simulink model "sgMdl_IO601_CAN_HS_Loopback"  (R2024b)
settings: Solver=FixedStepAuto  StartTime=0.0  StopTime=inf  RelTol=1e-3  EnableMultiTasking=on
undefined symbols (not defined in the file): CAN, MESSAGE
libraries: canmsglib x6, speedgoatlib_IO601 x5, slrealtimeutilitieslib x2, simulink x1
Description:
  | IO601 - CAN HS Loopback
settings Model: sg_rtwmakecfg_data=_sglibc_  ModifiedByFormat=Speedgoat  SimulationMode=external  ExtModeTrigDuration=100000  Creator=Speedgoat  LastModifiedBy=Speedgoat
settings SolverCC: ConcurrentTasks=on  AlgebraicLoopSolver=TrustRegion  PositivePriorityOrder=on  InsertRTBMode=Never (minimum delay)
settings DataIOCC: SaveFormat=StructureWithTime  ReturnWorkspaceOutputs=off
settings OptimizationCC: BlockReduction=off  OptimizeBlockIOStorage=off  BufferReuse=off  ReuseModelBlockBuffer=off  GlobalBufferReuse=off  ExpressionFolding=off  LocalBlockOutputs=off
settings DebuggingCC: TasksWithSamePriorityMsg=none  UnconnectedInputMsg=warning  UnconnectedOutputMsg=warning  UnconnectedLineMsg=warning  SFUnexpectedBacktrackingDiag=warning  SFNoUnconditionalDefaultTransitionDiag=warning  SFExecutionAtInitializationDiag=none  ArithmeticOperatorsInVariantConditions=warning
settings HardwareCC: ProdBitPerLong=64  ProdLongLongMode=on  ProdHWDeviceType=Intel->x86-64 (Linux 64)
settings ModelReferenceCC: EnableRefExpFcnMdlSchedulingChecks=on  PropagateSignalLabelsOutOfModel=off
settings SFSimCC: SimUseLocalCustomCode=off  CustomCodeUndefinedFunction=UseInterfaceOnly
settings RTWCC: Description=Speedgoat Real-Time Target Machine  SystemTargetFile=speedgoat.tlc  TemplateMakefile=slrealtime_default_tmf  RTWUseLocalCustomCode=off  Toolchain=Simulink Real-Time Toolchain  BuildConfiguration=Faster Runs  TargetLang=C++  GPUComputeCapability=3.5  DLArmComputeVersion=19.05
settings CodeAppCC: StateflowObjectComments=on
settings SimulinkRealTimeTargetCC: SubcomponentCodeInterfacePackaging=Reusable function  InstructionSetFMA=off  LogToMDFFile=off  SLRTFileLogMaxRuns=10  UseGCCFastMath=on
settings ConfigComp: CovMetricSettings=dw  CovSaveCumulativeToWorkspaceVar=on  CovSaveSingleToWorkspaceVar=on  CovExternalEMLEnable=off  CovBoundaryAbsTol=1.0e-5

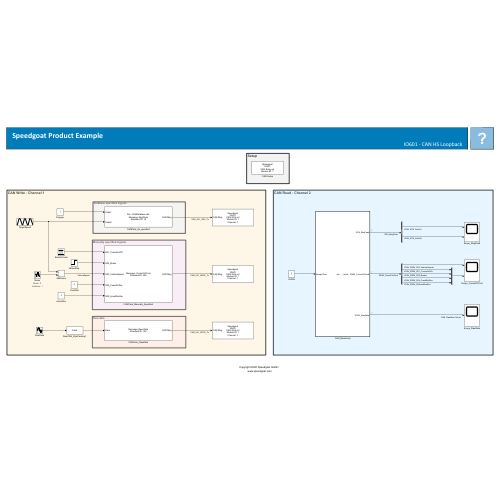
[thumbnail: Simulink's stored preview of the top-level diagram]
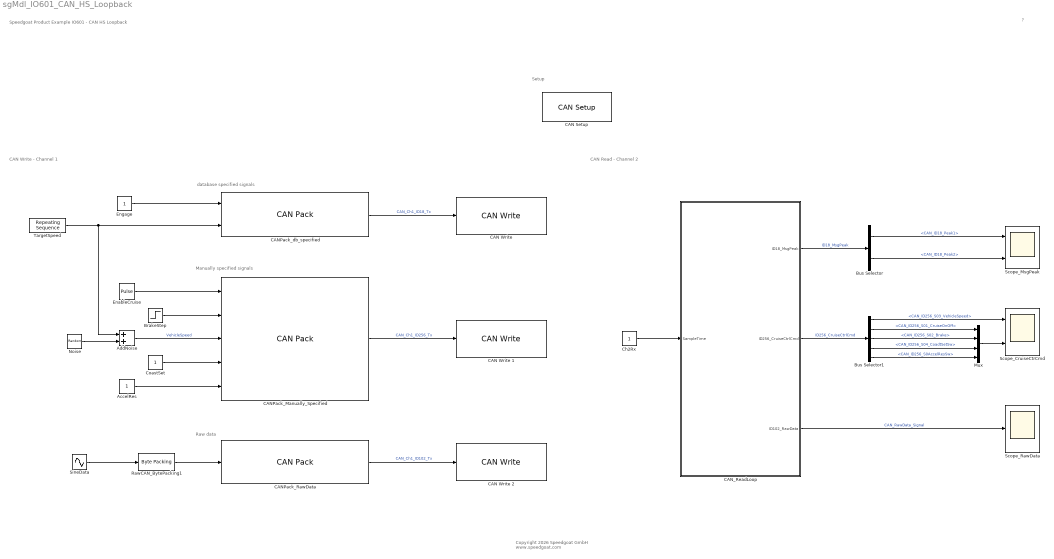
== system sgMdl_IO601_CAN_HS_Loopback ==
  note: CAN Write - Channel 1
  note: CAN Read - Channel 2
  note: database specified signals
  note: Manually specified signals
  note: Raw data
  note: Setup
  note: Speedgoat Product Example
      | IO601 - CAN HS Loopback
  note: ?
  note: Copyright 2026 Speedgoat GmbH
      |  www.speedgoat.com
  AccelRes : Constant  SampleTime=-1
  AddNoise : Sum
  BrakeStep : Step  Time=6  SampleTime=0.005
  Bus Selector : BusSelector  OutputSignals=CAN_ID18_Peak1,CAN_ID18_Peak2
  Bus Selector1 : BusSelector  OutputSignals=CAN_ID256_S03_VehicleSpeed,CAN_ID256_S01_CruiseOnOff,CAN_ID256_S02_Brake,CAN_ID256_S04_CoadtSetSw,CAN_ID256_S0AccelResSw
  CAN Setup : speedgoatlib_IO601/CAN Setup   id=1  initializationStructure=[]  terminationStructure=[]  pciSlot=-1  isCAN1Enalbe=on  operationModeCAN1=Highspeed  baudrateCAN1=1 MBaud  userDefinedBaudrateCAN1=[1 1 5 2]  standardAcceptanceMaskCAN1=[0,0,0,0]  extendenAcceptanceMaskCAN1=[0,0,0,0]  isCAN2Enable=on  operationModeCAN2=Highspeed  baudrateCAN2=1 MBaud  userDefinedBautrateCAN2=[1 1 5 2]  standardAcceptanceMaskCAN2=[0,0,0,0]  extendenAcceptanceMaskCAN2=[0,0,0,0]  isLINEndabled=off  LINRole=Master  LINBaudrate=20000  enhancedChecksumLIN=on
      settings: SourceProductName=Simulink Real-Time: Speedgoat I/O Blockset
  "CAN Write " : speedgoatlib_IO601/CAN/CAN Write   id=1  sampleTime=0.005  CANMessageDatatype=CAN-MESSAGE  CANPort=Port 1  isStatusOutputPortEnabled=off  PCISlot=-1  qtyWrtBlk=3
      settings: SourceProductName=Simulink Real-Time: Speedgoat I/O Blockset
  CAN Write 1 : speedgoatlib_IO601/CAN/CAN Write   id=1  sampleTime=0.005  CANMessageDatatype=CAN-MESSAGE  CANPort=Port 1  isStatusOutputPortEnabled=off  PCISlot=-1  qtyWrtBlk=3
      settings: SourceProductName=Simulink Real-Time: Speedgoat I/O Blockset
  CAN Write 2 : speedgoatlib_IO601/CAN/CAN Write   id=1  sampleTime=0.005  CANMessageDatatype=CAN-MESSAGE  CANPort=Port 1  isStatusOutputPortEnabled=off  PCISlot=-1  qtyWrtBlk=3
      settings: SourceProductName=Simulink Real-Time: Speedgoat I/O Blockset
  CANPack_Manually_Specified : canmsglib/CAN Pack  MsgList=(none)  MsgName=CruiseCtrlCmd  MsgIDType=Standard (11-bit identifier)  MsgIdentifier=256  CANIDInput=off  MsgLength=2  Remote=off  ApplyMinMax=off  BusOutput=off  SignalInfo={ 'S01_CruiseOnOff', '0', '1', 'LE', 'unsigned', 'Standard', '0', '1', '0', '0', '1'; 'S02_Brake', '1', '1', 'LE', 'unsigned', 'Standard', '0', '1', '0', '0', '1'; 'S03_VehicleSpeed', '4', '8', 'LE', 'unsigned', 'Standard', '0', '1', '0', '0', '255'; 'S04_CoastSetSw', '2', '1', 'LE', 'unsigned', 'Standard', '0', '1', '0', '0', '1'; 'S05_AccelResSw', '3', '1', 'LE', 'unsigned', 'Standard', '0', '1', '0', '0', '1' }
      settings: DataFormat=manually specified signals
  CANPack_RawData : canmsglib/CAN Pack  MsgList=(none)  MsgName=Raw Data  MsgIDType=Standard (11-bit identifier)  MsgIdentifier=102  CANIDInput=off  MsgLength=8  Remote=off  ApplyMinMax=off  BusOutput=off  SignalInfo={ 'Counter', '16', '7', 'LE', 'unsigned', 'Standard', '0', '1', '0', '-Inf', 'Inf'; 'Curve', '0', '16', 'LE', 'unsigned', 'Standard', '0', '0.1', '0', '0', '6500'; 'State', '23', '1', 'LE', 'unsigned', 'Standard', '0', '1', '0', '0', '1' }
      settings: DataFormat=raw data
  CANPack_db_specified : canmsglib/CAN Pack  CANdbFile=CANDatabase.dbc  MsgList=MsgPeak  MsgName=MsgPeak  MsgIDType=Standard (11-bit identifier)  MsgIdentifier=18  CANIDInput=off  MsgLength=4  Remote=off  ApplyMinMax=off  BusOutput=off  SignalInfo={'Peak1','0','8','LE','unsigned','Standard','0','1','0','0','255';'Peak2','8','8','LE','unsigned','Standard','0','1','0','0','255'}
      settings: DataFormat=CANdb specified signals
  CAN_ReadLoop : Subsystem  TreatAsAtomicUnit=on
  Ch2Rx : Constant  SampleTime=0.005
  CoastSet : Constant  SampleTime=-1
  EnableCruise : DiscretePulseGenerator  Period=200  PulseWidth=100  SampleTime=0.005
  Engage : Constant  SampleTime=-1
  Mux : Mux
  Noise : RandomNumber  SampleTime=0.005
      settings: AttributesFormatString=|
      | Mean: %<Mean>
      | Variance: %<Variance>
  RawCAN_BytePacking1 : slrealtimeutilitieslib/Byte Packing  MaskPackedDataType=uint8  MaskUnpackedDataTypes={'double'}  MaskAlignment=1
  Scope_CruiseCtrCmd : Scope  NumInputPorts=2
  Scope_MsgPeak : Scope  NumInputPorts=2
  Scope_RawData : Scope
  SineData : Sin  Amplitude=30  Bias=100  Frequency=2*pi  SampleTime=0.005
  TargetSpeed : simulink/Sources/Repeating Sequence  rep_seq_t=[0 1 4 6 10]  rep_seq_y=[0 0 50 50 0]
  wires:
  CANPack_RawData/1 -> CAN Write 2/1  "CAN_Ch1_ID102_Tx"
  RawCAN_BytePacking1/1 -> CANPack_RawData/1
  TargetSpeed/1 -> CANPack_db_specified/2, AddNoise/1
  Noise/1 -> AddNoise/2
  AddNoise/1 -> CANPack_Manually_Specified/3  "VehicleSpeed"
  BrakeStep/1 -> CANPack_Manually_Specified/2
  CANPack_db_specified/1 -> "CAN Write "/1  "CAN_Ch1_ID18_Tx"
  AccelRes/1 -> CANPack_Manually_Specified/5
  CANPack_Manually_Specified/1 -> CAN Write 1/1  "CAN_Ch1_ID256_Tx"
  CoastSet/1 -> CANPack_Manually_Specified/4
  Engage/1 -> CANPack_db_specified/1
  EnableCruise/1 -> CANPack_Manually_Specified/1
  SineData/1 -> RawCAN_BytePacking1/1
  CAN_ReadLoop/3(ID102_RawData) -> Scope_RawData/1  "CAN_RawData_Signal"
  CAN_ReadLoop/2(ID256_CruiseCtrlCmd) -> Bus Selector1/1  "ID256_CruiseCtrlCmd"
  Mux/1 -> Scope_CruiseCtrCmd/2
  CAN_ReadLoop/1(ID18_MsgPeak) -> Bus Selector/1  "ID18_MsgPeak"
  Bus Selector1/4 -> Mux/3  "<CAN_ID256_S04_CoadtSetSw>"
  Bus Selector/2 -> Scope_MsgPeak/2  "<CAN_ID18_Peak2>"
  Bus Selector1/3 -> Mux/2  "<CAN_ID256_S02_Brake>"
  Bus Selector1/2 -> Mux/1  "<CAN_ID256_S01_CruiseOnOff>"
  Bus Selector/1 -> Scope_MsgPeak/1  "<CAN_ID18_Peak1>"
  Ch2Rx/1 -> CAN_ReadLoop/1(SampleTime)
  Bus Selector1/1 -> Scope_CruiseCtrCmd/1  "<CAN_ID256_S03_VehicleSpeed>"
  Bus Selector1/5 -> Mux/4  "<CAN_ID256_S0AccelResSw>"

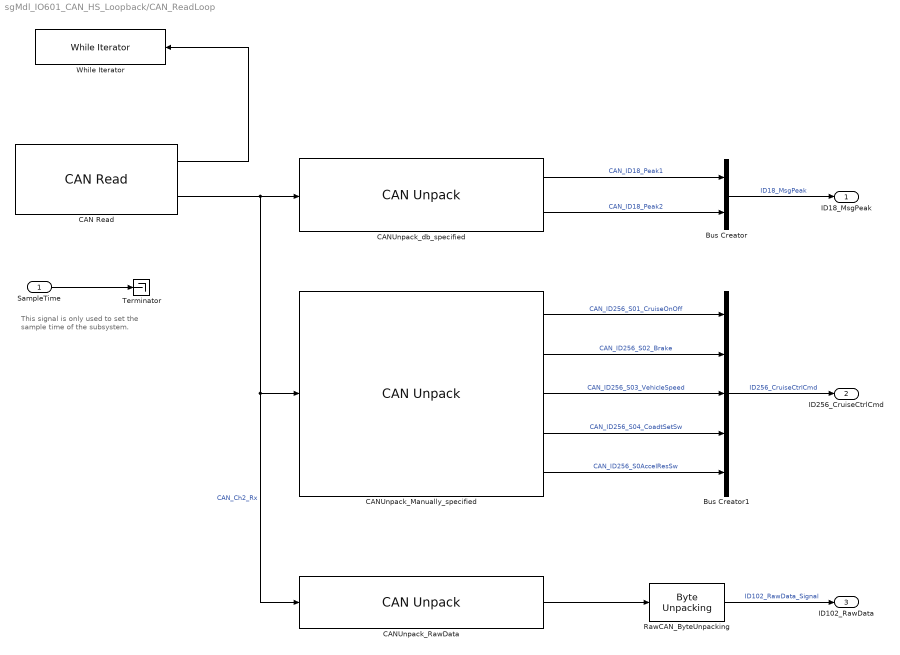
== system sgMdl_IO601_CAN_HS_Loopback/CAN_ReadLoop ==
  note: This signal is only used to set the sample time of the subsystem.
  SampleTime : Inport
  Bus Creator : BusCreator  Inputs=2
  Bus Creator1 : BusCreator  Inputs=5
  "CAN Read " : speedgoatlib_IO601/CAN/CAN Read   id=1  sampleTime=-1  CANMessageDatatype=CAN-MESSAGE  CANPort=Port 2  PCISlot=-1
      settings: SourceProductName=Simulink Real-Time: Speedgoat I/O Blockset
  CANUnpack_Manually_specified : canmsglib/CAN Unpack  MsgList=(none)  MsgName=CruiseCtrlCmd  MsgIDType=Standard (11-bit identifier)  MsgIdentifier=256  MsgLength=2  SignalInfo={ 'S01_CruiseOnOff', '0', '1', 'LE', 'unsigned', 'Standard', '0', '1', '0', '0', '1'; 'S02_Brake', '1', '1', 'LE', 'unsigned', 'Standard', '0', '1', '0', '0', '1'; 'S03_VehicleSpeed', '4', '8', 'LE', 'unsigned', 'Standard', '0', '1', '0', '0', '255'; 'S04_CoastSetSw', '2', '1', 'LE', 'unsigned', 'Standard', '0', '1', '0', '0', '1'; 'S05_AccelResSw', '3', '1', 'LE', 'unsigned', 'Standard', '0', '1', '0', '0', '1' }  IDPort=off  TimestampPort=off  ErrorPort=off  RemotePort=off  LengthPort=off  StatusPort=off  ApplyMinMax=off
  CANUnpack_RawData : canmsglib/CAN Unpack  MsgList=(none)  MsgName=Raw Data  MsgIDType=Standard (11-bit identifier)  MsgIdentifier=102  MsgLength=8  SignalInfo={ 'Counter', '16', '7', 'LE', 'unsigned', 'Standard', '0', '1', '0', '-Inf', 'Inf'; 'Curve', '0', '16', 'LE', 'unsigned', 'Standard', '0', '0.1', '0', '0', '6500'; 'State', '23', '1', 'LE', 'unsigned', 'Standard', '0', '1', '0', '0', '1' }  IDPort=off  TimestampPort=off  ErrorPort=off  RemotePort=off  LengthPort=off  StatusPort=off  ApplyMinMax=off
      settings: DataFormat=raw data
  CANUnpack_db_specified : canmsglib/CAN Unpack  CANdbFile=C:\svn\speedgoatlib\product_examples\IO601\IO601_files\CANDatabase.dbc  MsgList=MsgPeak  MsgName=MsgPeak  MsgIDType=Standard (11-bit identifier)  MsgIdentifier=18  MsgLength=4  SignalInfo={'Peak1','0','8','LE','unsigned','Standard','0','1','0','0','255';'Peak2','8','8','LE','unsigned','Standard','0','1','0','0','255'}  IDPort=off  TimestampPort=off  ErrorPort=off  RemotePort=off  LengthPort=off  StatusPort=off  ApplyMinMax=off
      settings: DataFormat=CANdb specified signals
  RawCAN_ByteUnpacking : slrealtimeutilitieslib/Byte Unpacking  MaskUnpackedDataTypes={'double'}  MaskUnpackedDataSizes={[1]}  MaskAlignment=1
  Terminator : Terminator
  While Iterator : WhileIterator  MaxIters=500  WhileBlockType=do-while
      settings: AttributesFormatString=|
      | ---
      | Max Numbers of iteration set to %<MaxIters>
      | This corresponds to the CAN HW buffer
  ID18_MsgPeak : Outport
  ID256_CruiseCtrlCmd : Outport  Port=2
  ID102_RawData : Outport  Port=3
  wires:
  "CAN Read "/1 -> While Iterator/1
  CANUnpack_db_specified/1 -> Bus Creator/1  "CAN_ID18_Peak1"
  CANUnpack_db_specified/2 -> Bus Creator/2  "CAN_ID18_Peak2"
  Bus Creator/1 -> ID18_MsgPeak/1  "ID18_MsgPeak"
  CANUnpack_Manually_specified/1 -> Bus Creator1/1  "CAN_ID256_S01_CruiseOnOff"
  CANUnpack_Manually_specified/2 -> Bus Creator1/2  "CAN_ID256_S02_Brake"
  CANUnpack_Manually_specified/3 -> Bus Creator1/3  "CAN_ID256_S03_VehicleSpeed"
  CANUnpack_Manually_specified/4 -> Bus Creator1/4  "CAN_ID256_S04_CoadtSetSw"
  CANUnpack_Manually_specified/5 -> Bus Creator1/5  "CAN_ID256_S0AccelResSw"
  Bus Creator1/1 -> ID256_CruiseCtrlCmd/1  "ID256_CruiseCtrlCmd"
  SampleTime/1 -> Terminator/1
  "CAN Read "/2 -> CANUnpack_RawData/1, CANUnpack_Manually_specified/1, CANUnpack_db_specified/1  "CAN_Ch2_Rx"
  CANUnpack_RawData/1 -> RawCAN_ByteUnpacking/1
  RawCAN_ByteUnpacking/1 -> ID102_RawData/1  "ID102_RawData_Signal"
